simulink model "Missile_Control_Loop"  (R2015b)
settings: Solver=VariableStepAuto  StartTime=0.0  StopTime=10.0  RelTol=1e-3
values from neighbouring files (symbols this model uses):
  G1 = G(1)    [Missile_linear.m]
  G2 = G(2)    [Missile_linear.m]
  V = 10    [Missile_linear.m]
undefined symbols (not defined in the file or in its folder): sigbuilder_block
settings Model: Creator=mathi  LastModifiedBy=mathi

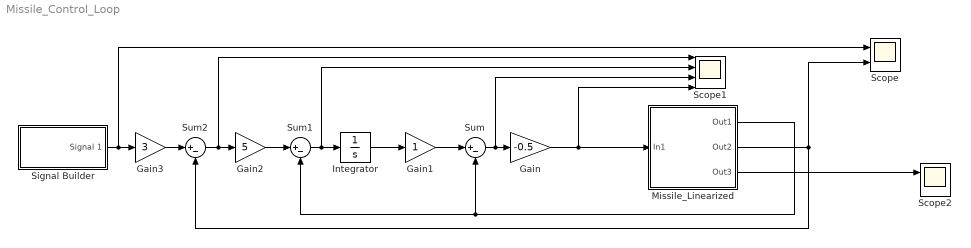
== system Missile_Control_Loop ==
  Gain : Gain  Gain=-0.5
  Gain1 : Gain
  Gain2 : Gain  Gain=5
  Gain3 : Gain  Gain=3
  Integrator : Integrator
  Missile_Linearized : Subsystem
      mask Display:
      | port_label('input',1,'\delta','texmode','on');
      | port_label('output',1,'\theta dot','texmode','on')
      | port_label('output',2,'A_z','texmode','on');
      | port_label('output',3,'\alpha dot','texmode','on');
  Scope : Scope  NumInputPorts=2
  Scope1 : Scope  NumInputPorts=4
  Scope2 : Scope  NumInputPorts=2
  Signal Builder : Subsystem  Tag=STV Subsys  LoadFcn=sigbuilder_block('load');  StartFcn=sigbuilder_block('start');  StopFcn=sigbuilder_block('stop');  ClipboardFcn=sigbuilder_block('clipboard');  mask(Sigbuilder block){}
      mask help: Simulink:masks:SigbuilderBlock_MD
      mask init:
      | if ~strcmp(get_param(bdroot(gcbh),'SimulationStatus'),'stopped') tuvar = sigbuilder_block('maskInit'); end
      settings: CopyFcn=sigbuilder_block('copy');  DeleteFcn=sigbuilder_block('delete');  ModelCloseFcn=sigbuilder_block('modelClose');  PreSaveFcn=sigbuilder_block('preSave');  PauseFcn=sigbuilder_block('pause');  ContinueFcn=sigbuilder_block('continue');  NameChangeFcn=sigbuilder_block('namechange');  OpenFcn=sigbuilder_block('open',[437.25 153 550.5 359.25 ]);  CloseFcn=sigbuilder_block('close');
      mask Display: plot(0, 0, 100, 100,[2, 2, 32, 32, 2], [68, 8, 8, 68, 68],[32, 2], [38, 38], [32, 19, 2],[53, 60, 44], [32, 17, 17, 2],[16, 16, 31, 31]);txt = getActiveGroup(gcbh);text(2, 100, txt,'verticalAlignment', 'top');
  Sum : Sum  Inputs=|+-
  Sum1 : Sum  Inputs=|+-
  Sum2 : Sum  Inputs=|+-
  wires:
  Gain/1 -> Missile_Linearized/1(In1), Scope1/4
  Sum1/1 -> Scope1/2, Integrator/1
  Sum2/1 -> Scope1/1, Gain2/1
  Gain3/1 -> Sum2/1
  Gain2/1 -> Sum1/1
  Integrator/1 -> Gain1/1
  Gain1/1 -> Sum/1
  Missile_Linearized/1(Out1) -> Sum1/2, Sum/2
  Missile_Linearized/2(Out2) -> Sum2/2, Scope/2
  Signal Builder/1(Signal 1) -> Scope/1, Gain3/1
  Sum/1 -> Scope1/3, Gain/1
  Missile_Linearized/3(Out3) -> Scope2/1

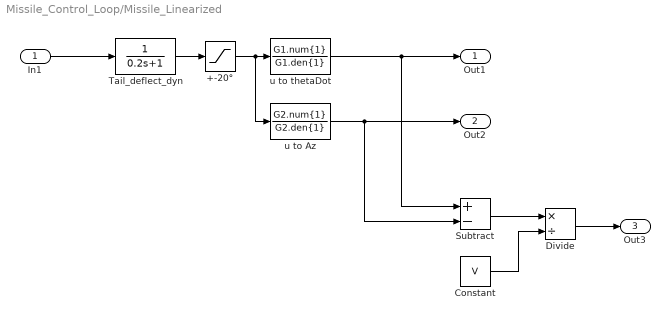
== system Missile_Control_Loop/Missile_Linearized ==
  In1 : Inport
  +-20° : Saturate  UpperLimit=0.35  LowerLimit=-0.35
  Constant : Constant  Value=V
  Divide : Product  Inputs=*/
  Subtract : Sum  Inputs=+-
  Tail_deflect_dyn : TransferFcn  Denominator=[0.2 1]
  u to Az : TransferFcn  Numerator=G2.num{1}  Denominator=G2.den{1}
  u to thetaDot : TransferFcn  Numerator=G1.num{1}  Denominator=G1.den{1}
  Out1 : Outport
  Out2 : Outport  Port=2
  Out3 : Outport  Port=3
  wires:
  In1/1 -> Tail_deflect_dyn/1
  u to Az/1 -> Subtract/2, Out2/1
  u to thetaDot/1 -> Subtract/1, Out1/1
  Tail_deflect_dyn/1 -> +-20°/1
  +-20°/1 -> u to Az/1, u to thetaDot/1
  Subtract/1 -> Divide/1
  Constant/1 -> Divide/2
  Divide/1 -> Out3/1

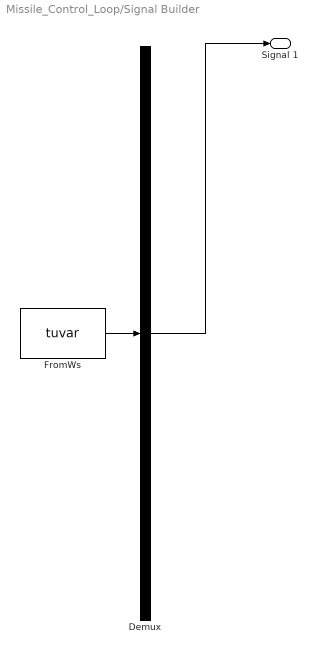
== system Missile_Control_Loop/Signal Builder ==
  Demux : Demux  Tag=STV Demux  Outputs=1
  FromWs : FromWorkspace  Tag=STV FromWs  VariableName=tuvar  SampleTime=0
      SigBuilderData=|
      | common.afterFinalStr = 'Extrapolate'
      | common.sampleTime = 0
      | dataSet.timeRange = [0 10]
      | dataSet.name = 'Group 1'
      | sbobj.Groups.Name = 'Group 1'
      | sbobj.Groups.Signals.Name = 'Signal 1'
      | sbobj.Groups.Signals.XData = [0 1.6 1.6 6.08 6.08 10]
      | sbobj.Groups.Signals.YData = [0 0 1 1 0 0]
  Signal 1 : Outport  Tag=STV Outport
  wires:
  Demux/1 -> Signal 1/1
  FromWs/1 -> Demux/1
